simulink model "bquad"  (Simulink 7.2)
settings: Solver=ode45  StartTime=0.0  StopTime=100.0  RelTol=1e-4
libraries: cstblocks x10
settings Model: Creator=rana  LastModifiedBy=rana  ExtModeTrigMode=oneshot  ExtModeArmWhenConnect=off  ExtModeAutoUpdateStatusClock=off
settings DataIOCC: LimitDataPoints=off
settings OptimizationCC: BlockReduction=off  BooleanDataType=off  InlineInvariantSignals=on  InitFltsAndDblsToZero=on
settings DebuggingCC: SaveWithParameterizedLinksMsg=none  SignalResolutionControl=TryResolveAllWithWarning  SolverPrmCheckMsg=none  MultiTaskDSMMsg=warning  MultiTaskCondExecSysMsg=none  UnconnectedInputMsg=none  UnconnectedOutputMsg=none  StrictBusMsg=None
settings HardwareCC: TargetUnknown=on
settings RTWCC: IncludeERTFirstTime=on
settings GRTTargetCC: TargetFcnLib=ansi_tfl_tmw.mat  ModelReferenceCompliant=off  MatFileLogging=off

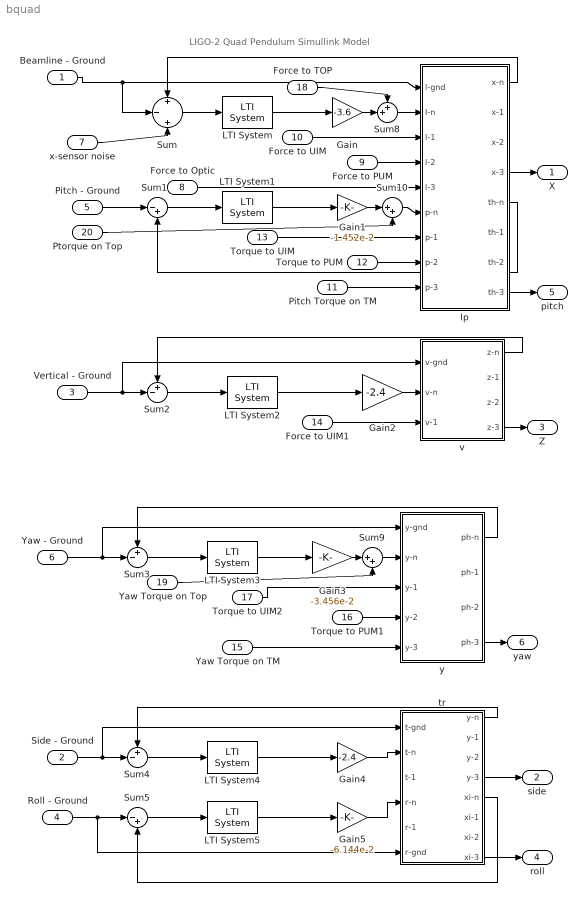
== system bquad ==
  note: LIGO-2 Quad Pendulum Simullink Model
  Beamline - Ground : Inport  OutDataType=sfix(16)  OutScaling=2^0
  Side - Ground : Inport  Port=2  OutDataType=sfix(16)  OutScaling=2^0
  Vertical - Ground : Inport  Port=3  OutDataType=sfix(16)  OutScaling=2^0
  Roll - Ground : Inport  Port=4  OutDataType=sfix(16)  OutScaling=2^0
  Pitch - Ground : Inport  Port=5  OutDataType=sfix(16)  OutScaling=2^0
  Yaw - Ground : Inport  Port=6  OutDataType=sfix(16)  OutScaling=2^0
  x-sensor noise : Inport  Port=7  OutDataType=sfix(16)  OutScaling=2^0
  Force to Optic : Inport  Port=8  OutDataType=sfix(16)  OutScaling=2^0
  Force to PUM : Inport  Port=9  OutDataType=sfix(16)  OutScaling=2^0
  Force to UIM : Inport  Port=10  OutDataType=sfix(16)  OutScaling=2^0
  Pitch Torque on TM : Inport  Port=11  OutDataType=sfix(16)  OutScaling=2^0
  Torque to PUM : Inport  Port=12  OutDataType=sfix(16)  OutScaling=2^0
  Torque to UIM : Inport  Port=13  OutDataType=sfix(16)  OutScaling=2^0
  Force to UIM1 : Inport  Port=14  OutDataType=sfix(16)  OutScaling=2^0
  Yaw Torque on TM : Inport  Port=15  OutDataType=sfix(16)  OutScaling=2^0
  Torque to PUM1 : Inport  Port=16  OutDataType=sfix(16)  OutScaling=2^0
  Torque to UIM2 : Inport  Port=17  OutDataType=sfix(16)  OutScaling=2^0
  Force to TOP : Inport  Port=18  OutDataType=sfix(16)  OutScaling=2^0
  Yaw Torque on Top : Inport  Port=19  OutDataType=sfix(16)  OutScaling=2^0
  Ptorque on Top : Inport  Port=20  OutDataType=sfix(16)  OutScaling=2^0
  Gain : Gain  Gain=-3.6  ParameterDataType=sfix(16)  ParameterScaling=2^0  OutDataType=sfix(16)  OutScaling=2^0  OutDataTypeStr=Inherit: Same as input  ParamDataTypeStr=Inherit: Same as input
  Gain1 : Gain  Gain=-1.452e-2  ParameterDataType=sfix(16)  ParameterScaling=2^0  OutDataType=sfix(16)  OutScaling=2^0  OutDataTypeStr=Inherit: Same as input  ParamDataTypeStr=Inherit: Same as input
  Gain2 : Gain  Gain=-2.4  ParameterDataType=sfix(16)  ParameterScaling=2^0  OutDataType=sfix(16)  OutScaling=2^0  OutDataTypeStr=Inherit: Same as input  ParamDataTypeStr=Inherit: Same as input
  Gain3 : Gain  Gain=-3.456e-2  ParameterDataType=sfix(16)  ParameterScaling=2^0  OutDataType=sfix(16)  OutScaling=2^0  OutDataTypeStr=Inherit: Same as input  ParamDataTypeStr=Inherit: Same as input
  Gain4 : Gain  Gain=-2.4  ParameterDataType=sfix(16)  ParameterScaling=2^0  OutDataType=sfix(16)  OutScaling=2^0  OutDataTypeStr=Inherit: Same as input  ParamDataTypeStr=Inherit: Same as input
  Gain5 : Gain  Gain=-6.144e-2  ParameterDataType=sfix(16)  ParameterScaling=2^0  OutDataType=sfix(16)  OutScaling=2^0  OutDataTypeStr=Inherit: Same as input  ParamDataTypeStr=Inherit: Same as input
  LTI System : cstblocks/LTI System  SystemSampleTime=-1  sys=ldamp  IC=[]
  LTI System1 : cstblocks/LTI System  SystemSampleTime=-1  sys=pdamp  IC=[]
  LTI System2 : cstblocks/LTI System  SystemSampleTime=-1  sys=vdamp  IC=[]
  LTI System3 : cstblocks/LTI System  SystemSampleTime=-1  sys=ydamp  IC=[]
  LTI System4 : cstblocks/LTI System  SystemSampleTime=-1  sys=tdamp  IC=[]
  LTI System5 : cstblocks/LTI System  SystemSampleTime=-1  sys=rdamp  IC=[]
  Sum : Sum  Inputs=+|-|+  OutDataType=sfix(16)  OutScaling=2^0  InputSameDT=on  OutDataTypeStr=Inherit: Same as first input
  Sum1 : Sum  Inputs=|-+  OutDataType=sfix(16)  OutScaling=2^0  InputSameDT=on  OutDataTypeStr=Inherit: Same as first input
  Sum10 : Sum  Inputs=|++  OutDataType=sfix(16)  OutScaling=2^0  InputSameDT=on  OutDataTypeStr=Inherit: Same as first input
  Sum2 : Sum  Inputs=+-|  OutDataType=sfix(16)  OutScaling=2^0  InputSameDT=on  OutDataTypeStr=Inherit: Same as first input
  Sum3 : Sum  Inputs=+-|  OutDataType=sfix(16)  OutScaling=2^0  InputSameDT=on  OutDataTypeStr=Inherit: Same as first input
  Sum4 : Sum  Inputs=+-|  OutDataType=sfix(16)  OutScaling=2^0  InputSameDT=on  OutDataTypeStr=Inherit: Same as first input
  Sum5 : Sum  Inputs=|-+  OutDataType=sfix(16)  OutScaling=2^0  InputSameDT=on  OutDataTypeStr=Inherit: Same as first input
  Sum8 : Sum  Inputs=++|  OutDataType=sfix(16)  OutScaling=2^0  InputSameDT=on  OutDataTypeStr=Inherit: Same as first input
  Sum9 : Sum  Inputs=|++  OutDataType=sfix(16)  OutScaling=2^0  InputSameDT=on  OutDataTypeStr=Inherit: Same as first input
  lp : Subsystem
  tr : Subsystem
  v : Subsystem
  y : Subsystem
  X : Outport  OutDataType=sfix(16)  OutScaling=2^0
  side : Outport  Port=2  OutDataType=sfix(16)  OutScaling=2^0
  Z : Outport  Port=3  OutDataType=sfix(16)  OutScaling=2^0
  roll : Outport  Port=4  OutDataType=sfix(16)  OutScaling=2^0
  pitch : Outport  Port=5  OutDataType=sfix(16)  OutScaling=2^0
  yaw : Outport  Port=6  OutDataType=sfix(16)  OutScaling=2^0
  wires:
  Gain2/1 -> v/2(v-n)
  Gain4/1 -> tr/2(t-n)
  Gain5/1 -> tr/4(r-n)
  Gain1/1 -> Sum10/1
  y/1(ph-n) -> Sum3/1
  tr/5(xi-n) -> Sum5/2
  tr/1(y-n) -> Sum4/1
  lp/5(th-n) -> Sum1/2
  lp/1(x-n) -> Sum/1
  LTI System/1 -> Gain/1
  Sum1/1 -> LTI System1/1
  Sum3/1 -> LTI System3/1
  Sum4/1 -> LTI System4/1
  Sum5/1 -> LTI System5/1
  v/1(z-n) -> Sum2/1
  Sum/1 -> LTI System/1
  Sum2/1 -> LTI System2/1
  Beamline - Ground/1 -> lp/1(l-gnd), Sum/2
  Pitch - Ground/1 -> Sum1/1
  Vertical - Ground/1 -> Sum2/2, v/1(v-gnd)
  Yaw - Ground/1 -> Sum3/2, y/1(y-gnd)
  Side - Ground/1 -> Sum4/2, tr/1(t-gnd)
  Roll - Ground/1 -> Sum5/1, tr/6(r-gnd)
  lp/4(x-3) -> X/1
  tr/4(y-3) -> side/1
  v/4(z-3) -> Z/1
  tr/8(xi-3) -> roll/1
  lp/8(th-3) -> pitch/1
  y/4(ph-3) -> yaw/1
  LTI System1/1 -> Gain1/1
  LTI System2/1 -> Gain2/1
  LTI System3/1 -> Gain3/1
  LTI System4/1 -> Gain4/1
  LTI System5/1 -> Gain5/1
  x-sensor noise/1 -> Sum/3
  Force to PUM/1 -> lp/4(l-2)
  Force to UIM/1 -> lp/3(l-1)
  Pitch Torque on TM/1 -> lp/9(p-3)
  Torque to PUM/1 -> lp/8(p-2)
  Torque to UIM/1 -> lp/7(p-1)
  Force to Optic/1 -> lp/5(l-3)
  Force to UIM1/1 -> v/3(v-1)
  Torque to UIM2/1 -> y/3(y-1)
  Torque to PUM1/1 -> y/4(y-2)
  Yaw Torque on TM/1 -> y/5(y-3)
  Gain/1 -> Sum8/2
  Sum8/1 -> lp/2(I-n)
  Force to TOP/1 -> Sum8/1
  Gain3/1 -> Sum9/1
  Sum9/1 -> y/2(y-n)
  Yaw Torque on Top/1 -> Sum9/2
  Sum10/1 -> lp/6(p-n)
  Ptorque on Top/1 -> Sum10/2

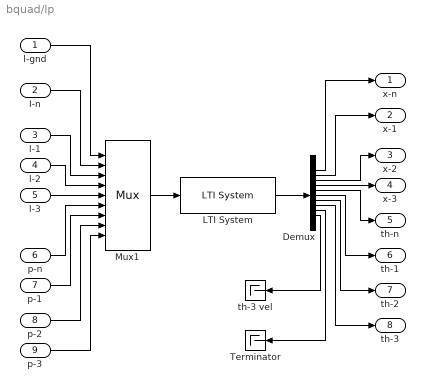
== system bquad/lp ==
  l-gnd : Inport  OutDataType=sfix(16)  OutScaling=2^0
  I-n : Inport  Port=2  OutDataType=sfix(16)  OutScaling=2^0
  l-1 : Inport  Port=3  OutDataType=sfix(16)  OutScaling=2^0
  l-2 : Inport  Port=4  OutDataType=sfix(16)  OutScaling=2^0
  l-3 : Inport  Port=5  OutDataType=sfix(16)  OutScaling=2^0
  p-n : Inport  Port=6  OutDataType=sfix(16)  OutScaling=2^0
  p-1 : Inport  Port=7  OutDataType=sfix(16)  OutScaling=2^0
  p-2 : Inport  Port=8  OutDataType=sfix(16)  OutScaling=2^0
  p-3 : Inport  Port=9  OutDataType=sfix(16)  OutScaling=2^0
  Demux : Demux  Outputs=10
  LTI System : cstblocks/LTI System  SystemSampleTime=-1  sys=lpe  IC=[0]
  Mux1 : Mux  Inputs=9
      settings: DisplayOption=signals
  Terminator : Terminator
  th-3 vel : Terminator
  x-n : Outport  OutDataType=sfix(16)  OutScaling=2^0
  x-1 : Outport  Port=2  OutDataType=sfix(16)  OutScaling=2^0
  x-2 : Outport  Port=3  OutDataType=sfix(16)  OutScaling=2^0
  x-3 : Outport  Port=4  OutDataType=sfix(16)  OutScaling=2^0
  th-n : Outport  Port=5  OutDataType=sfix(16)  OutScaling=2^0
  th-1 : Outport  Port=6  OutDataType=sfix(16)  OutScaling=2^0
  th-2 : Outport  Port=7  OutDataType=sfix(16)  OutScaling=2^0
  th-3 : Outport  Port=8  OutDataType=sfix(16)  OutScaling=2^0
  wires:
  Mux1/1 -> LTI System/1
  LTI System/1 -> Demux/1
  Demux/1 -> x-n/1
  Demux/2 -> x-1/1
  Demux/3 -> x-2/1
  Demux/4 -> x-3/1
  Demux/5 -> th-n/1
  Demux/6 -> th-1/1
  Demux/7 -> th-2/1
  Demux/8 -> th-3/1
  l-gnd/1 -> Mux1/1
  I-n/1 -> Mux1/2
  l-1/1 -> Mux1/3
  l-2/1 -> Mux1/4
  l-3/1 -> Mux1/5
  p-n/1 -> Mux1/6
  p-1/1 -> Mux1/7
  p-2/1 -> Mux1/8
  p-3/1 -> Mux1/9
  Demux/9 -> Terminator/1
  Demux/10 -> th-3 vel/1

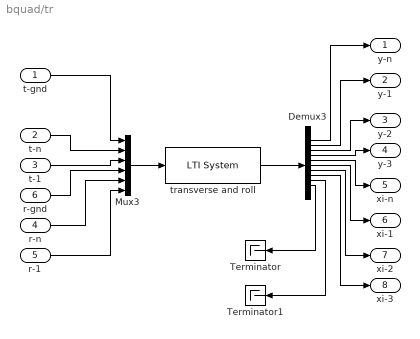
== system bquad/tr ==
  t-gnd : Inport  OutDataType=sfix(16)  OutScaling=2^0
  t-n : Inport  Port=2  OutDataType=sfix(16)  OutScaling=2^0
  t-1 : Inport  Port=3  OutDataType=sfix(16)  OutScaling=2^0
  r-n : Inport  Port=4  OutDataType=sfix(16)  OutScaling=2^0
  r-1 : Inport  Port=5  OutDataType=sfix(16)  OutScaling=2^0
  r-gnd : Inport  Port=6  OutDataType=sfix(16)  OutScaling=2^0
  Demux3 : Demux  Outputs=10
  Mux3 : Mux  Inputs=6
  Terminator : Terminator
  Terminator1 : Terminator
  transverse and roll : cstblocks/LTI System  SystemSampleTime=-1  sys=trer  IC=[0]
  y-n : Outport  OutDataType=sfix(16)  OutScaling=2^0
  y-1 : Outport  Port=2  OutDataType=sfix(16)  OutScaling=2^0
  y-2 : Outport  Port=3  OutDataType=sfix(16)  OutScaling=2^0
  y-3 : Outport  Port=4  OutDataType=sfix(16)  OutScaling=2^0
  xi-n : Outport  Port=5  OutDataType=sfix(16)  OutScaling=2^0
  xi-1 : Outport  Port=6  OutDataType=sfix(16)  OutScaling=2^0
  xi-2 : Outport  Port=7  OutDataType=sfix(16)  OutScaling=2^0
  xi-3 : Outport  Port=8  OutDataType=sfix(16)  OutScaling=2^0
  wires:
  Mux3/1 -> transverse and roll/1
  transverse and roll/1 -> Demux3/1
  Demux3/1 -> y-n/1
  Demux3/2 -> y-1/1
  Demux3/3 -> y-2/1
  Demux3/4 -> y-3/1
  Demux3/5 -> xi-n/1
  Demux3/6 -> xi-1/1
  Demux3/7 -> xi-2/1
  Demux3/8 -> xi-3/1
  t-gnd/1 -> Mux3/1
  t-n/1 -> Mux3/2
  t-1/1 -> Mux3/3
  r-1/1 -> Mux3/6
  r-n/1 -> Mux3/5
  r-gnd/1 -> Mux3/4
  Demux3/9 -> Terminator1/1
  Demux3/10 -> Terminator/1

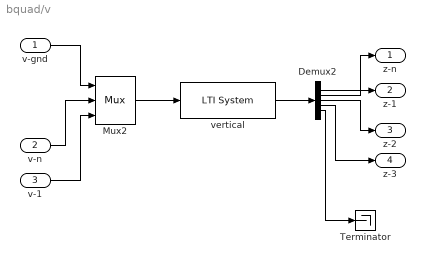
== system bquad/v ==
  v-gnd : Inport  OutDataType=sfix(16)  OutScaling=2^0
  v-n : Inport  Port=2  OutDataType=sfix(16)  OutScaling=2^0
  v-1 : Inport  Port=3  OutDataType=sfix(16)  OutScaling=2^0
  Demux2 : Demux  Outputs=5
  Mux2 : Mux  Inputs=3
      settings: DisplayOption=signals
  Terminator : Terminator
  vertical : cstblocks/LTI System  SystemSampleTime=-1  sys=ve  IC=[0]
  z-n : Outport  OutDataType=sfix(16)  OutScaling=2^0
  z-1 : Outport  Port=2  OutDataType=sfix(16)  OutScaling=2^0
  z-2 : Outport  Port=3  OutDataType=sfix(16)  OutScaling=2^0
  z-3 : Outport  Port=4  OutDataType=sfix(16)  OutScaling=2^0
  wires:
  Mux2/1 -> vertical/1
  vertical/1 -> Demux2/1
  v-gnd/1 -> Mux2/1
  Demux2/1 -> z-n/1
  Demux2/2 -> z-1/1
  Demux2/3 -> z-2/1
  Demux2/4 -> z-3/1
  v-1/1 -> Mux2/3
  v-n/1 -> Mux2/2
  Demux2/5 -> Terminator/1

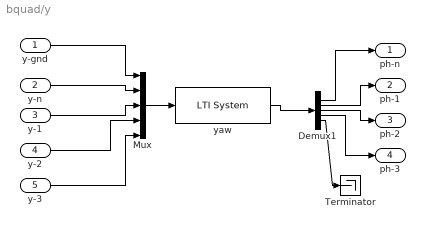
== system bquad/y ==
  y-gnd : Inport  OutDataType=sfix(16)  OutScaling=2^0
  y-n : Inport  Port=2  OutDataType=sfix(16)  OutScaling=2^0
  y-1 : Inport  Port=3  OutDataType=sfix(16)  OutScaling=2^0
  y-2 : Inport  Port=4  OutDataType=sfix(16)  OutScaling=2^0
  y-3 : Inport  Port=5  OutDataType=sfix(16)  OutScaling=2^0
  Demux1 : Demux  Outputs=5
  Mux : Mux  Inputs=5
  Terminator : Terminator
  yaw : cstblocks/LTI System  SystemSampleTime=-1  sys=ye  IC=[0]
  ph-n : Outport  OutDataType=sfix(16)  OutScaling=2^0
  ph-1 : Outport  Port=2  OutDataType=sfix(16)  OutScaling=2^0
  ph-2 : Outport  Port=3  OutDataType=sfix(16)  OutScaling=2^0
  ph-3 : Outport  Port=4  OutDataType=sfix(16)  OutScaling=2^0
  wires:
  y-gnd/1 -> Mux/1
  Mux/1 -> yaw/1
  yaw/1 -> Demux1/1
  Demux1/1 -> ph-n/1
  Demux1/2 -> ph-1/1
  Demux1/3 -> ph-2/1
  Demux1/4 -> ph-3/1
  y-3/1 -> Mux/5
  y-2/1 -> Mux/4
  y-1/1 -> Mux/3
  y-n/1 -> Mux/2
  Demux1/5 -> Terminator/1
